simulink model "Sim_PA_DDPG_4drone"  (R2025a)
settings: Solver=ode1  StartTime=0.0  StopTime=Tf  FixedStep=Ts_Sim  RelTol=1e-3
undefined symbols (not defined in the file): control_noise, p_IC, phi_IC, phi_limit, pqr_Limit, psi_dsr, psi_IC, psi_limit, q_IC, r_IC, saturation_logic, state_noise, theta_IC, theta_limit, Ts_Sim, u_IC, uvw_Limit, v_IC, w_IC, wind_logic, x_IC, xy_Limit, y_IC, z_IC, z_Limit
libraries: rllib x8
(part 1 of 2)
settings Model: Creator=nt488543  LastModifiedBy=re606359

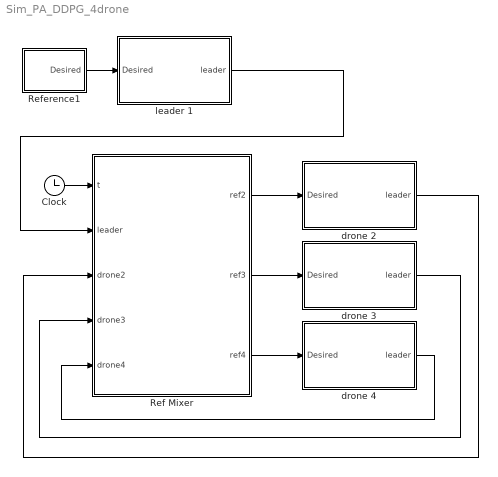
== system Sim_PA_DDPG_4drone ==
  Clock : Clock
  Ref Mixer : MATLAB Function  TreatAsAtomicUnit=on
  Reference1 : Subsystem
  drone 2 : Subsystem
  drone 3 : Subsystem
  drone 4 : Subsystem
  leader 1 : Subsystem
  wires:
  Reference1/1(Desired) -> leader 1/1(Desired)
  Clock/1 -> Ref Mixer/1(t)
  leader 1/1(leader) -> Ref Mixer/2(leader)
  Ref Mixer/1(ref2) -> drone 2/1(Desired)
  Ref Mixer/2(ref3) -> drone 3/1(Desired)
  Ref Mixer/3(ref4) -> drone 4/1(Desired)
  drone 2/1(leader) -> Ref Mixer/3(drone2)
  drone 3/1(leader) -> Ref Mixer/4(drone3)
  drone 4/1(leader) -> Ref Mixer/5(drone4)

== system Sim_PA_DDPG_4drone/Reference1 ==
  Clock1 : Clock
  Mux : Mux  Inputs=6
  Position Reference Signal : MATLAB Function  TreatAsAtomicUnit=on
  To Workspace : ToWorkspace  VariableName=X_ref  SampleTime=Ts_Sim
  Desired : Outport
  wires:
  Position Reference Signal/2(y_desired) -> Mux/2  "y_desired"
  Position Reference Signal/4(xdot_desired) -> Mux/4  "u_desired"
  Position Reference Signal/6(zdot_desired) -> Mux/6  "w_desired"
  Clock1/1 -> Position Reference Signal/1(t)
  Position Reference Signal/3(z_desired) -> Mux/3  "z_desired"
  Position Reference Signal/1(x_desired) -> Mux/1  "x_desired"
  Position Reference Signal/5(ydot_desired) -> Mux/5  "v_desired"
  Mux/1 -> To Workspace/1, Desired/1  "Desired"

== system Sim_PA_DDPG_4drone/drone 2 ==
  note: Inner Loop
  Desired : Inport
  Attitude DDPG : Subsystem
  Drone Dynamics : Subsystem
  Position DDPG : Subsystem
  System Solver : Subsystem
  leader : Outport
  wires:
  Drone Dynamics/2(Actual Angle & its Rate) -> Attitude DDPG/2(Actual Angle)
  System Solver/1(Ang Ref) -> Attitude DDPG/1(Angle Reference)
  Attitude DDPG/1(Tau) -> Drone Dynamics/1(Tau)  "Tau"
  System Solver/2(ft) -> Drone Dynamics/2(ft)
  Desired/1 -> Position DDPG/1(Desired)
  Position DDPG/1(uvw Dot) -> System Solver/1(uvw Dot)
  Drone Dynamics/1(Actual Position & Velocity) -> Position DDPG/2(Actual Position & Velocity), leader/1  "Outer Loop"

== system Sim_PA_DDPG_4drone/drone 3 ==
  note: Inner Loop
  Desired : Inport
  Attitude DDPG : Subsystem
  Drone Dynamics : Subsystem
  Position DDPG : Subsystem
  System Solver : Subsystem
  leader : Outport
  wires:
  Drone Dynamics/1(Actual Position & Velocity) -> leader/1, Position DDPG/2(Actual Position & Velocity)  "Outer Loop"
  Position DDPG/1(uvw Dot) -> System Solver/1(uvw Dot)
  Desired/1 -> Position DDPG/1(Desired)
  System Solver/2(ft) -> Drone Dynamics/2(ft)
  Attitude DDPG/1(Tau) -> Drone Dynamics/1(Tau)  "Tau"
  System Solver/1(Ang Ref) -> Attitude DDPG/1(Angle Reference)
  Drone Dynamics/2(Actual Angle & its Rate) -> Attitude DDPG/2(Actual Angle)

== system Sim_PA_DDPG_4drone/drone 4 ==
  note: Inner Loop
  Desired : Inport
  Attitude DDPG : Subsystem
  Drone Dynamics : Subsystem
  Position DDPG : Subsystem
  System Solver : Subsystem
  leader : Outport
  wires:
  Drone Dynamics/2(Actual Angle & its Rate) -> Attitude DDPG/2(Actual Angle)
  System Solver/1(Ang Ref) -> Attitude DDPG/1(Angle Reference)
  Attitude DDPG/1(Tau) -> Drone Dynamics/1(Tau)  "Tau"
  System Solver/2(ft) -> Drone Dynamics/2(ft)
  Desired/1 -> Position DDPG/1(Desired)
  Position DDPG/1(uvw Dot) -> System Solver/1(uvw Dot)
  Drone Dynamics/1(Actual Position & Velocity) -> Position DDPG/2(Actual Position & Velocity), leader/1  "Outer Loop"

== system Sim_PA_DDPG_4drone/leader 1 ==
  note: Inner Loop
  Desired : Inport
  Attitude DDPG : Subsystem
  Drone Dynamics : Subsystem
  Position DDPG : Subsystem
  System Solver : Subsystem
  leader : Outport
  wires:
  Drone Dynamics/1(Actual Position & Velocity) -> leader/1, Position DDPG/2(Actual Position & Velocity)  "Outer Loop"
  Position DDPG/1(uvw Dot) -> System Solver/1(uvw Dot)
  Desired/1 -> Position DDPG/1(Desired)
  System Solver/2(ft) -> Drone Dynamics/2(ft)
  Attitude DDPG/1(Tau) -> Drone Dynamics/1(Tau)  "Tau"
  System Solver/1(Ang Ref) -> Attitude DDPG/1(Angle Reference)
  Drone Dynamics/2(Actual Angle & its Rate) -> Attitude DDPG/2(Actual Angle)

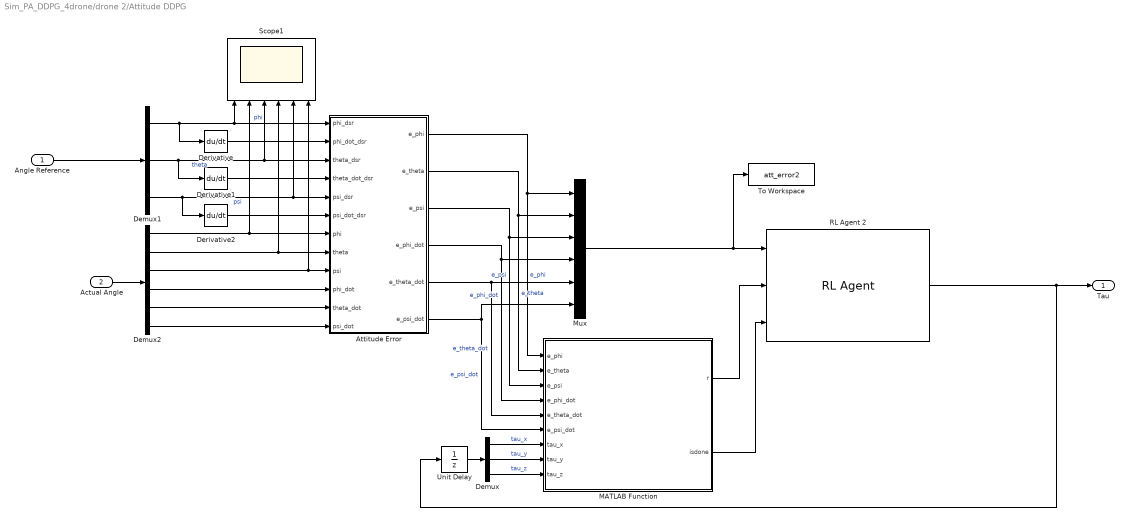
== system Sim_PA_DDPG_4drone/drone 2/Attitude DDPG ==
  Angle Reference : Inport
  Actual Angle : Inport  Port=2
  Attitude Error : MATLAB Function  TreatAsAtomicUnit=on
  Demux : Demux  Outputs=3
  Demux1 : Demux  Outputs=3
  Demux2 : Demux  Outputs=6
  Derivative : Derivative
  Derivative1 : Derivative
  Derivative2 : Derivative
  MATLAB Function : MATLAB Function  TreatAsAtomicUnit=on
  Mux : Mux  Inputs=6
  RL Agent 2 : rllib/RL Agent  Agent=agent2  ExternalActionAsInput=off  ProvideLastAction=off  ProvideCumRwd=off  TreatAsDirectFeedthrough=on  UseStrictObservationDataTypes=off
  Scope1 : Scope  NumInputPorts=6
      settings: ActiveDisplayYMinimum=-0.08548920227975057  ActiveDisplayYMaximum=0.079586119310867051  DataLoggingVariableName=ScopeData6
  To Workspace : ToWorkspace  VariableName=att_error2  SampleTime=Ts_Sim
  Unit Delay : UnitDelay  SampleTime=Ts_Sim  HasFrameUpgradeWarning=on
  Tau : Outport
  wires:
  Derivative2/1 -> Attitude Error/6(psi_dot_dsr)
  Derivative1/1 -> Attitude Error/4(theta_dot_dsr)
  Derivative/1 -> Attitude Error/2(phi_dot_dsr)
  Angle Reference/1 -> Demux1/1
  Demux1/2 -> Scope1/3, Attitude Error/3(theta_dsr), Derivative1/1  "theta"
  Demux1/3 -> Scope1/5, Attitude Error/5(psi_dsr), Derivative2/1  "psi"
  Demux1/1 -> Scope1/1, Attitude Error/1(phi_dsr), Derivative/1  "phi"
  Unit Delay/1 -> Demux/1
  Actual Angle/1 -> Demux2/1
  Demux2/6 -> Attitude Error/12(psi_dot)
  Demux2/5 -> Attitude Error/11(theta_dot)
  Demux2/4 -> Attitude Error/10(phi_dot)
  Demux2/3 -> Scope1/6, Attitude Error/9(psi)
  Demux2/2 -> Attitude Error/8(theta), Scope1/4
  Demux2/1 -> Attitude Error/7(phi), Scope1/2
  RL Agent 2/1 -> Tau/1, Unit Delay/1
  Demux/3 -> MATLAB Function/9(tau_z)  "tau_z"
  Demux/2 -> MATLAB Function/8(tau_y)  "tau_y"
  Demux/1 -> MATLAB Function/7(tau_x)  "tau_x"
  MATLAB Function/2(isdone) -> RL Agent 2/3
  Attitude Error/6(e_psi_dot) -> Mux/6, MATLAB Function/6(e_psi_dot)  "e_psi_dot"
  Attitude Error/5(e_theta_dot) -> Mux/5, MATLAB Function/5(e_theta_dot)  "e_theta_dot"
  Attitude Error/4(e_phi_dot) -> MATLAB Function/4(e_phi_dot), Mux/4  "e_phi_dot"
  Attitude Error/3(e_psi) -> MATLAB Function/3(e_psi), Mux/3  "e_psi"
  Attitude Error/2(e_theta) -> MATLAB Function/2(e_theta), Mux/2  "e_theta"
  Attitude Error/1(e_phi) -> MATLAB Function/1(e_phi), Mux/1  "e_phi"
  Mux/1 -> RL Agent 2/1, To Workspace/1
  MATLAB Function/1(r) -> RL Agent 2/2

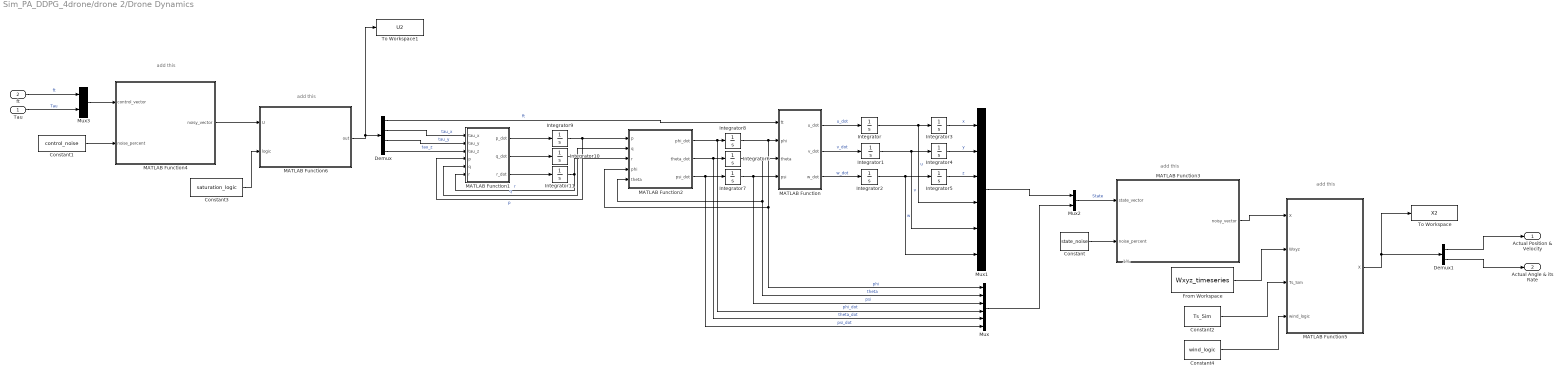
== system Sim_PA_DDPG_4drone/drone 2/Drone Dynamics ==
  note: add this
  note: add this
  note: add this
  note: 1%
  note: add this
  Tau : Inport
  ft : Inport  Port=2
  Constant : Constant  Value=state_noise  SampleTime=Ts_Sim
  Constant1 : Constant  Value=control_noise
  Constant2 : Constant  Value=Ts_Sim
  Constant3 : Constant  Value=saturation_logic  SampleTime=Ts_Sim
  Constant4 : Constant  Value=wind_logic
  Demux : Demux
  Demux1 : Demux  Outputs=2
  From Workspace : FromWorkspace  VariableName=Wxyz_timeseries  SampleTime=Ts_Sim
  Integrator : Integrator  InitialCondition=u_IC  UpperSaturationLimit=uvw_Limit  LowerSaturationLimit=-uvw_Limit
  Integrator1 : Integrator  InitialCondition=v_IC  UpperSaturationLimit=uvw_Limit  LowerSaturationLimit=-uvw_Limit
  Integrator10 : Integrator  InitialCondition=q_IC  UpperSaturationLimit=pqr_Limit  LowerSaturationLimit=-pqr_Limit
  Integrator11 : Integrator  InitialCondition=r_IC  UpperSaturationLimit=pqr_Limit  LowerSaturationLimit=-pqr_Limit
  Integrator2 : Integrator  InitialCondition=w_IC  UpperSaturationLimit=uvw_Limit  LowerSaturationLimit=-uvw_Limit
  Integrator3 : Integrator  InitialCondition=x_IC  UpperSaturationLimit=xy_Limit  LowerSaturationLimit=-xy_Limit
  Integrator4 : Integrator  InitialCondition=y_IC  UpperSaturationLimit=xy_Limit  LowerSaturationLimit=-xy_Limit
  Integrator5 : Integrator  InitialCondition=z_IC  UpperSaturationLimit=z_Limit  LowerSaturationLimit=-z_Limit
  Integrator6 : Integrator  InitialCondition=theta_IC  UpperSaturationLimit=theta_limit  LowerSaturationLimit=-theta_limit  WrappedStateUpperValue=pi/2  WrappedStateLowerValue=-pi/2
  Integrator7 : Integrator  InitialCondition=psi_IC  UpperSaturationLimit=psi_limit  LowerSaturationLimit=-psi_limit
  Integrator8 : Integrator  InitialCondition=phi_IC  UpperSaturationLimit=phi_limit  LowerSaturationLimit=-phi_limit
  Integrator9 : Integrator  InitialCondition=p_IC  UpperSaturationLimit=pqr_Limit  LowerSaturationLimit=-pqr_Limit
  MATLAB Function : MATLAB Function  TreatAsAtomicUnit=on
  MATLAB Function1 : MATLAB Function  TreatAsAtomicUnit=on
  MATLAB Function2 : MATLAB Function  TreatAsAtomicUnit=on
  MATLAB Function3 : MATLAB Function  TreatAsAtomicUnit=on
  MATLAB Function4 : MATLAB Function  TreatAsAtomicUnit=on
  MATLAB Function5 : MATLAB Function  TreatAsAtomicUnit=on
  MATLAB Function6 : MATLAB Function  TreatAsAtomicUnit=on
  Mux : Mux  Inputs=6
  Mux1 : Mux  Inputs=6
  Mux2 : Mux  Inputs=2
  Mux3 : Mux  Inputs=2
  To Workspace : ToWorkspace  VariableName=X2  SampleTime=Ts_Sim
  To Workspace1 : ToWorkspace  VariableName=U2  SampleTime=Ts_Sim
  Actual Position & Velocity : Outport
  Actual Angle & its Rate : Outport  Port=2
  wires:
  Constant4/1 -> MATLAB Function5/4(wind_logic)
  Constant3/1 -> MATLAB Function6/2(logic)
  MATLAB Function6/1(out) -> Demux/1, To Workspace1/1
  MATLAB Function5/1(X) -> Demux1/1, To Workspace/1
  Constant2/1 -> MATLAB Function5/3(Ts_Sim)
  Demux1/1 -> Actual Position & Velocity/1
  Demux1/2 -> Actual Angle & its Rate/1
  From Workspace/1 -> MATLAB Function5/2(Wxyz)
  Demux/1 -> MATLAB Function/1(ft)  "ft"
  MATLAB Function4/1(noisy_vector) -> MATLAB Function6/1(U)
  Constant1/1 -> MATLAB Function4/2(noise_percent)
  Mux3/1 -> MATLAB Function4/1(control_vector)
  Constant/1 -> MATLAB Function3/2(noise_percent)
  Mux1/1 -> Mux2/1
  MATLAB Function3/1(noisy_vector) -> MATLAB Function5/1("X ")
  Mux2/1 -> MATLAB Function3/1(state_vector)  "State"
  MATLAB Function2/3(psi_dot) -> Integrator7/1, Mux/6  "psi_dot"
  MATLAB Function2/2(theta_dot) -> Integrator6/1, Mux/5  "theta_dot"
  MATLAB Function2/1(phi_dot) -> Integrator8/1, Mux/4  "phi_dot"
  Demux/2 -> MATLAB Function1/1(tau_x)  "tau_x"
  MATLAB Function1/2(q_dot) -> Integrator10/1
  MATLAB Function/2(v_dot) -> Integrator1/1  "v_dot"
  MATLAB Function/1(u_dot) -> Integrator/1  "u_dot"
  MATLAB Function/3(w_dot) -> Integrator2/1  "w_dot"
  Mux/1 -> Mux2/2
  Demux/4 -> MATLAB Function1/3(tau_z)  "tau_z"
  Integrator10/1 -> MATLAB Function1/5(q), MATLAB Function2/2(q)  "q"
  Integrator6/1 -> MATLAB Function2/5(theta), Mux/2, MATLAB Function/3(theta)  "theta"
  Integrator8/1 -> MATLAB Function/2(phi), MATLAB Function2/4(phi), Mux/1  "phi"
  Integrator7/1 -> MATLAB Function/4(psi), Mux/3  "psi"
  Tau/1 -> Mux3/2  "Tau"
  Integrator/1 -> Integrator3/1, Mux1/4  "u"
  Integrator2/1 -> Integrator5/1, Mux1/6  "w"
  Integrator11/1 -> MATLAB Function2/3(r), MATLAB Function1/6(r)  "r"
  Integrator9/1 -> MATLAB Function2/1(p), MATLAB Function1/4(p)  "p"
  Demux/3 -> MATLAB Function1/2(tau_y)  "tau_y"
  ft/1 -> Mux3/1  "ft"
  Integrator1/1 -> Integrator4/1, Mux1/5  "v"
  Integrator5/1 -> Mux1/3  "z"
  Integrator3/1 -> Mux1/1  "x"
  MATLAB Function1/1(p_dot) -> Integrator9/1
  MATLAB Function1/3(r_dot) -> Integrator11/1
  Integrator4/1 -> Mux1/2  "y"

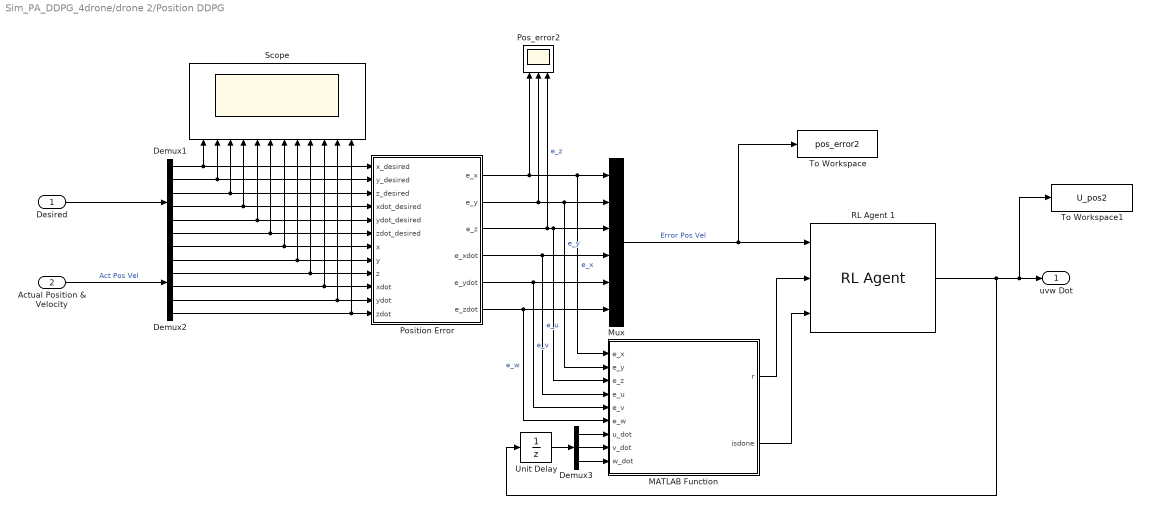
== system Sim_PA_DDPG_4drone/drone 2/Position DDPG ==
  Desired : Inport
  Actual Position & Velocity : Inport  Port=2
  Demux1 : Demux  Outputs=6
  Demux2 : Demux  Outputs=6
  Demux3 : Demux  Outputs=3
  MATLAB Function : MATLAB Function  TreatAsAtomicUnit=on
  Mux : Mux  Inputs=6
  Pos_error2 : Scope  NumInputPorts=3
      settings: ActiveDisplayYMinimum=-19.835443512065805  ActiveDisplayYMaximum=10.081140709923583  DataLoggingVariableName=Error2
  Position Error : MATLAB Function  TreatAsAtomicUnit=on
  RL Agent 1 : rllib/RL Agent  Agent=agent  ExternalActionAsInput=off  ProvideLastAction=off  ProvideCumRwd=off  TreatAsDirectFeedthrough=on  UseStrictObservationDataTypes=off
  Scope : Scope  NumInputPorts=12
      settings: ActiveDisplayYMinimum=-58.33042936718266  ActiveDisplayYMaximum=11.607599309056914  DataLoggingVariableName=Difference
  To Workspace : ToWorkspace  VariableName=pos_error2  SampleTime=Ts_Sim
  To Workspace1 : ToWorkspace  VariableName=U_pos2  SampleTime=Ts_Sim
  Unit Delay : UnitDelay  SampleTime=Ts_Sim  HasFrameUpgradeWarning=on
  uvw Dot : Outport
  wires:
  Unit Delay/1 -> Demux3/1
  Demux3/3 -> MATLAB Function/9(w_dot)
  Demux3/2 -> MATLAB Function/8(v_dot)
  Demux3/1 -> MATLAB Function/7(u_dot)
  Actual Position & Velocity/1 -> Demux2/1  "Act Pos Vel"
  Demux2/6 -> Position Error/12(zdot), Scope/12
  Demux2/5 -> Scope/11, Position Error/11(ydot)
  Demux2/4 -> Scope/10, Position Error/10(xdot)
  Demux2/3 -> Scope/9, Position Error/9(z)
  Demux2/2 -> Scope/8, Position Error/8(y)
  Demux2/1 -> Scope/7, Position Error/7(x)
  Desired/1 -> Demux1/1
  Demux1/6 -> Scope/6, Position Error/6(zdot_desired)
  Demux1/5 -> Scope/5, Position Error/5(ydot_desired)
  Demux1/4 -> Scope/4, Position Error/4(xdot_desired)
  Demux1/3 -> Scope/3, Position Error/3(z_desired)
  Demux1/2 -> Scope/2, Position Error/2(y_desired)
  Demux1/1 -> Scope/1, Position Error/1(x_desired)
  MATLAB Function/2(isdone) -> RL Agent 1/3
  Position Error/6(e_zdot) -> Mux/6, MATLAB Function/6(e_w)  "e_w"
  Position Error/5(e_ydot) -> Mux/5, MATLAB Function/5(e_v)  "e_v"
  Position Error/4(e_xdot) -> Mux/4, MATLAB Function/4(e_u)  "e_u"
  RL Agent 1/1 -> Unit Delay/1, uvw Dot/1, To Workspace1/1
  Mux/1 -> RL Agent 1/1, To Workspace/1  "Error Pos Vel"
  MATLAB Function/1(r) -> RL Agent 1/2
  Position Error/3(e_z) -> Pos_error2/3, MATLAB Function/3(e_z), Mux/3  "e_z"
  Position Error/1(e_x) -> Pos_error2/1, Mux/1, MATLAB Function/1(e_x)  "e_x"
  Position Error/2(e_y) -> Pos_error2/2, Mux/2, MATLAB Function/2(e_y)  "e_y"

== system Sim_PA_DDPG_4drone/drone 2/System Solver ==
  uvw Dot : Inport
  Clock : Clock
  Constant : Constant  Value=psi_dsr
  Demux : Demux  Outputs=3
  Mux : Mux  Inputs=3
  Scope : Scope
      settings: ActiveDisplayYMinimum=5.5477079741609581  ActiveDisplayYMaximum=13.965080226414941
  System Solver : MATLAB Function  TreatAsAtomicUnit=on
  Ang Ref : Outport
  ft : Outport  Port=2
  wires:
  Constant/1 -> System Solver/5("r_yaw ")
  uvw Dot/1 -> Demux/1
  Mux/1 -> Ang Ref/1  "Ang Ref"
  Clock/1 -> System Solver/4(Ts)
  System Solver/4(ft) -> Scope/1, ft/1  "ft"
  Demux/3 -> System Solver/3(u3)
  System Solver/1(roll) -> Mux/1
  Demux/2 -> System Solver/2(u2)
  System Solver/3(r_yaw) -> Mux/3
  Demux/1 -> System Solver/1(u1)
  System Solver/2(pitch) -> Mux/2

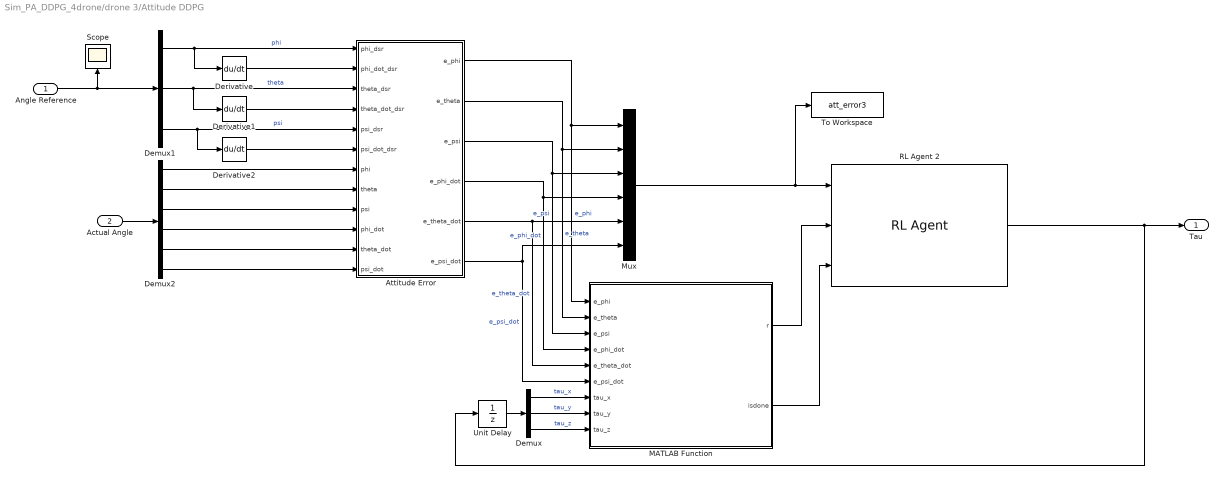
== system Sim_PA_DDPG_4drone/drone 3/Attitude DDPG ==
  Angle Reference : Inport
  Actual Angle : Inport  Port=2
  Attitude Error : MATLAB Function  TreatAsAtomicUnit=on
  Demux : Demux  Outputs=3
  Demux1 : Demux  Outputs=3
  Demux2 : Demux  Outputs=6
  Derivative : Derivative
  Derivative1 : Derivative
  Derivative2 : Derivative
  MATLAB Function : MATLAB Function  TreatAsAtomicUnit=on
  Mux : Mux  Inputs=6
  RL Agent 2 : rllib/RL Agent  Agent=agent2  ExternalActionAsInput=off  ProvideLastAction=off  ProvideCumRwd=off  TreatAsDirectFeedthrough=on  UseStrictObservationDataTypes=off
  Scope : Scope
      settings: ActiveDisplayYMinimum=-0.07573  ActiveDisplayYMaximum=0.06612  DataLoggingVariableName=ScopeData5
  To Workspace : ToWorkspace  VariableName=att_error3  SampleTime=Ts_Sim
  Unit Delay : UnitDelay  SampleTime=Ts_Sim  HasFrameUpgradeWarning=on
  Tau : Outport
  wires:
  MATLAB Function/1(r) -> RL Agent 2/2
  Mux/1 -> To Workspace/1, RL Agent 2/1
  Attitude Error/1(e_phi) -> Mux/1, MATLAB Function/1(e_phi)  "e_phi"
  Attitude Error/2(e_theta) -> Mux/2, MATLAB Function/2(e_theta)  "e_theta"
  Attitude Error/3(e_psi) -> Mux/3, MATLAB Function/3(e_psi)  "e_psi"
  Attitude Error/4(e_phi_dot) -> Mux/4, MATLAB Function/4(e_phi_dot)  "e_phi_dot"
  Attitude Error/5(e_theta_dot) -> MATLAB Function/5(e_theta_dot), Mux/5  "e_theta_dot"
  Attitude Error/6(e_psi_dot) -> MATLAB Function/6(e_psi_dot), Mux/6  "e_psi_dot"
  MATLAB Function/2(isdone) -> RL Agent 2/3
  Demux/1 -> MATLAB Function/7(tau_x)  "tau_x"
  Demux/2 -> MATLAB Function/8(tau_y)  "tau_y"
  Demux/3 -> MATLAB Function/9(tau_z)  "tau_z"
  RL Agent 2/1 -> Unit Delay/1, Tau/1
  Demux2/1 -> Attitude Error/7(phi)
  Demux2/2 -> Attitude Error/8(theta)
  Demux2/3 -> Attitude Error/9(psi)
  Demux2/4 -> Attitude Error/10(phi_dot)
  Demux2/5 -> Attitude Error/11(theta_dot)
  Demux2/6 -> Attitude Error/12(psi_dot)
  Actual Angle/1 -> Demux2/1
  Unit Delay/1 -> Demux/1
  Demux1/1 -> Derivative/1, Attitude Error/1(phi_dsr)  "phi"
  Demux1/3 -> Derivative2/1, Attitude Error/5(psi_dsr)  "psi"
  Demux1/2 -> Derivative1/1, Attitude Error/3(theta_dsr)  "theta"
  Angle Reference/1 -> Demux1/1, Scope/1
  Derivative/1 -> Attitude Error/2(phi_dot_dsr)
  Derivative1/1 -> Attitude Error/4(theta_dot_dsr)
  Derivative2/1 -> Attitude Error/6(psi_dot_dsr)

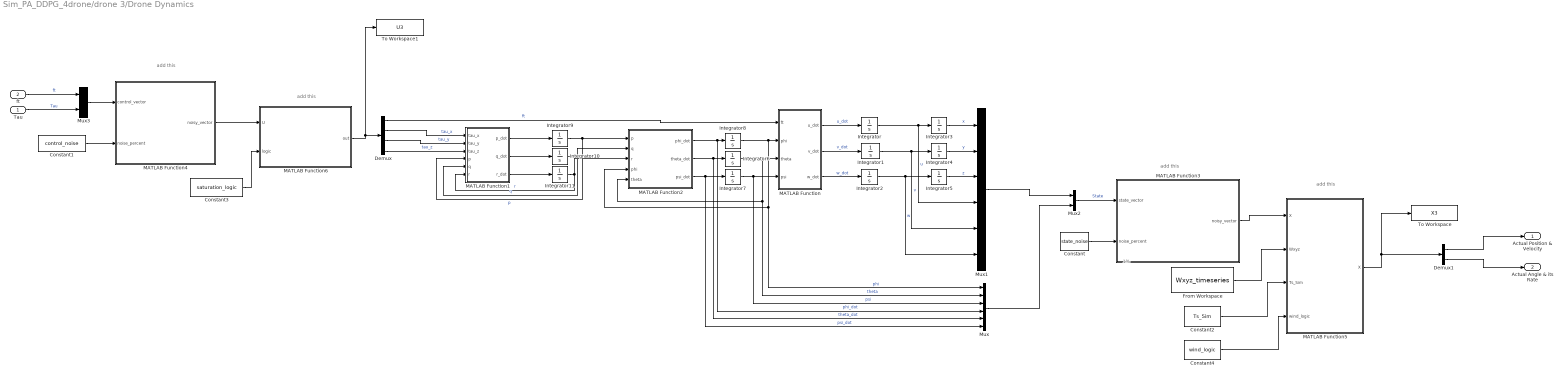
== system Sim_PA_DDPG_4drone/drone 3/Drone Dynamics ==
  note: add this
  note: 1%
  note: add this
  note: add this
  note: add this
  Tau : Inport
  ft : Inport  Port=2
  Constant : Constant  Value=state_noise  SampleTime=Ts_Sim
  Constant1 : Constant  Value=control_noise
  Constant2 : Constant  Value=Ts_Sim
  Constant3 : Constant  Value=saturation_logic  SampleTime=Ts_Sim
  Constant4 : Constant  Value=wind_logic
  Demux : Demux
  Demux1 : Demux  Outputs=2
  From Workspace : FromWorkspace  VariableName=Wxyz_timeseries  SampleTime=Ts_Sim
  Integrator : Integrator  InitialCondition=u_IC  UpperSaturationLimit=uvw_Limit  LowerSaturationLimit=-uvw_Limit
  Integrator1 : Integrator  InitialCondition=v_IC  UpperSaturationLimit=uvw_Limit  LowerSaturationLimit=-uvw_Limit
  Integrator10 : Integrator  InitialCondition=q_IC  UpperSaturationLimit=pqr_Limit  LowerSaturationLimit=-pqr_Limit
  Integrator11 : Integrator  InitialCondition=r_IC  UpperSaturationLimit=pqr_Limit  LowerSaturationLimit=-pqr_Limit
  Integrator2 : Integrator  InitialCondition=w_IC  UpperSaturationLimit=uvw_Limit  LowerSaturationLimit=-uvw_Limit
  Integrator3 : Integrator  InitialCondition=x_IC  UpperSaturationLimit=xy_Limit  LowerSaturationLimit=-xy_Limit
  Integrator4 : Integrator  InitialCondition=y_IC  UpperSaturationLimit=xy_Limit  LowerSaturationLimit=-xy_Limit
  Integrator5 : Integrator  InitialCondition=z_IC  UpperSaturationLimit=z_Limit  LowerSaturationLimit=-z_Limit
  Integrator6 : Integrator  InitialCondition=theta_IC  UpperSaturationLimit=theta_limit  LowerSaturationLimit=-theta_limit  WrappedStateUpperValue=pi/2  WrappedStateLowerValue=-pi/2
  Integrator7 : Integrator  InitialCondition=psi_IC  UpperSaturationLimit=psi_limit  LowerSaturationLimit=-psi_limit
  Integrator8 : Integrator  InitialCondition=phi_IC  UpperSaturationLimit=phi_limit  LowerSaturationLimit=-phi_limit
  Integrator9 : Integrator  InitialCondition=p_IC  UpperSaturationLimit=pqr_Limit  LowerSaturationLimit=-pqr_Limit
  MATLAB Function : MATLAB Function  TreatAsAtomicUnit=on
  MATLAB Function1 : MATLAB Function  TreatAsAtomicUnit=on
  MATLAB Function2 : MATLAB Function  TreatAsAtomicUnit=on
  MATLAB Function3 : MATLAB Function  TreatAsAtomicUnit=on
  MATLAB Function4 : MATLAB Function  TreatAsAtomicUnit=on
  MATLAB Function5 : MATLAB Function  TreatAsAtomicUnit=on
  MATLAB Function6 : MATLAB Function  TreatAsAtomicUnit=on
  Mux : Mux  Inputs=6
  Mux1 : Mux  Inputs=6
  Mux2 : Mux  Inputs=2
  Mux3 : Mux  Inputs=2
  To Workspace : ToWorkspace  VariableName=X3  SampleTime=Ts_Sim
  To Workspace1 : ToWorkspace  VariableName=U3  SampleTime=Ts_Sim
  Actual Position & Velocity : Outport
  Actual Angle & its Rate : Outport  Port=2
  wires:
  Integrator4/1 -> Mux1/2  "y"
  MATLAB Function1/3(r_dot) -> Integrator11/1
  MATLAB Function1/1(p_dot) -> Integrator9/1
  Integrator3/1 -> Mux1/1  "x"
  Integrator5/1 -> Mux1/3  "z"
  Integrator1/1 -> Mux1/5, Integrator4/1  "v"
  ft/1 -> Mux3/1  "ft"
  Demux/3 -> MATLAB Function1/2(tau_y)  "tau_y"
  Integrator9/1 -> MATLAB Function1/4(p), MATLAB Function2/1(p)  "p"
  Integrator11/1 -> MATLAB Function1/6(r), MATLAB Function2/3(r)  "r"
  Integrator2/1 -> Mux1/6, Integrator5/1  "w"
  Integrator/1 -> Mux1/4, Integrator3/1  "u"
  Tau/1 -> Mux3/2  "Tau"
  Integrator7/1 -> Mux/3, MATLAB Function/4(psi)  "psi"
  Integrator8/1 -> Mux/1, MATLAB Function2/4(phi), MATLAB Function/2(phi)  "phi"
  Integrator6/1 -> MATLAB Function/3(theta), Mux/2, MATLAB Function2/5(theta)  "theta"
  Integrator10/1 -> MATLAB Function2/2(q), MATLAB Function1/5(q)  "q"
  Demux/4 -> MATLAB Function1/3(tau_z)  "tau_z"
  Mux/1 -> Mux2/2
  MATLAB Function/3(w_dot) -> Integrator2/1  "w_dot"
  MATLAB Function/1(u_dot) -> Integrator/1  "u_dot"
  MATLAB Function/2(v_dot) -> Integrator1/1  "v_dot"
  MATLAB Function1/2(q_dot) -> Integrator10/1
  Demux/2 -> MATLAB Function1/1(tau_x)  "tau_x"
  MATLAB Function2/1(phi_dot) -> Mux/4, Integrator8/1  "phi_dot"
  MATLAB Function2/2(theta_dot) -> Mux/5, Integrator6/1  "theta_dot"
  MATLAB Function2/3(psi_dot) -> Mux/6, Integrator7/1  "psi_dot"
  Mux2/1 -> MATLAB Function3/1(state_vector)  "State"
  MATLAB Function3/1(noisy_vector) -> MATLAB Function5/1("X ")
  Mux1/1 -> Mux2/1
  Constant/1 -> MATLAB Function3/2(noise_percent)
  Mux3/1 -> MATLAB Function4/1(control_vector)
  Constant1/1 -> MATLAB Function4/2(noise_percent)
  MATLAB Function4/1(noisy_vector) -> MATLAB Function6/1(U)
  Demux/1 -> MATLAB Function/1(ft)  "ft"
  From Workspace/1 -> MATLAB Function5/2(Wxyz)
  Demux1/2 -> Actual Angle & its Rate/1
  Demux1/1 -> Actual Position & Velocity/1
  Constant2/1 -> MATLAB Function5/3(Ts_Sim)
  MATLAB Function5/1(X) -> To Workspace/1, Demux1/1
  MATLAB Function6/1(out) -> To Workspace1/1, Demux/1
  Constant3/1 -> MATLAB Function6/2(logic)
  Constant4/1 -> MATLAB Function5/4(wind_logic)

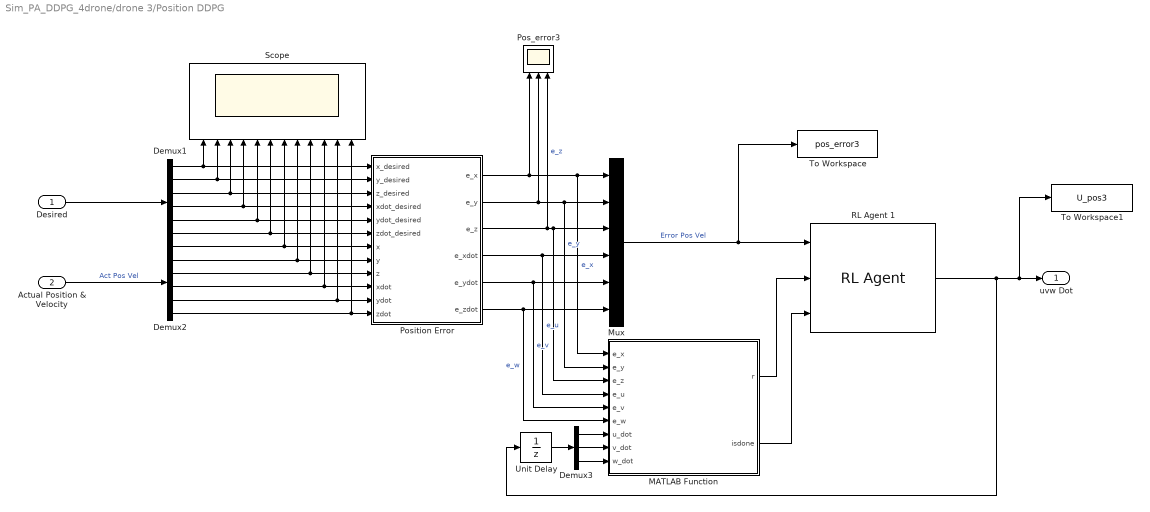
== system Sim_PA_DDPG_4drone/drone 3/Position DDPG ==
  Desired : Inport
  Actual Position & Velocity : Inport  Port=2
  Demux1 : Demux  Outputs=6
  Demux2 : Demux  Outputs=6
  Demux3 : Demux  Outputs=3
  MATLAB Function : MATLAB Function  TreatAsAtomicUnit=on
  Mux : Mux  Inputs=6
  Pos_error3 : Scope  NumInputPorts=3
      settings: ActiveDisplayYMinimum=-26.259185565275498  ActiveDisplayYMaximum=15.642824664105513  DataLoggingVariableName=Error3
  Position Error : MATLAB Function  TreatAsAtomicUnit=on
  RL Agent 1 : rllib/RL Agent  Agent=agent  ExternalActionAsInput=off  ProvideLastAction=off  ProvideCumRwd=off  TreatAsDirectFeedthrough=on  UseStrictObservationDataTypes=off
  Scope : Scope  NumInputPorts=12
      settings: ActiveDisplayYMinimum=-64.8105630976365  ActiveDisplayYMaximum=12.296113517917625  DataLoggingVariableName=Difference
  To Workspace : ToWorkspace  VariableName=pos_error3  SampleTime=Ts_Sim
  To Workspace1 : ToWorkspace  VariableName=U_pos3  SampleTime=Ts_Sim
  Unit Delay : UnitDelay  SampleTime=Ts_Sim  HasFrameUpgradeWarning=on
  uvw Dot : Outport
  wires:
  MATLAB Function/1(r) -> RL Agent 1/2
  Mux/1 -> To Workspace/1, RL Agent 1/1  "Error Pos Vel"
  RL Agent 1/1 -> To Workspace1/1, uvw Dot/1, Unit Delay/1
  Position Error/4(e_xdot) -> MATLAB Function/4(e_u), Mux/4  "e_u"
  Position Error/5(e_ydot) -> MATLAB Function/5(e_v), Mux/5  "e_v"
  Position Error/6(e_zdot) -> MATLAB Function/6(e_w), Mux/6  "e_w"
  MATLAB Function/2(isdone) -> RL Agent 1/3
  Demux1/1 -> Position Error/1(x_desired), Scope/1
  Demux1/2 -> Position Error/2(y_desired), Scope/2
  Demux1/3 -> Position Error/3(z_desired), Scope/3
  Demux1/4 -> Position Error/4(xdot_desired), Scope/4
  Demux1/5 -> Position Error/5(ydot_desired), Scope/5
  Demux1/6 -> Position Error/6(zdot_desired), Scope/6
  Desired/1 -> Demux1/1
  Demux2/1 -> Position Error/7(x), Scope/7
  Demux2/2 -> Position Error/8(y), Scope/8
  Demux2/3 -> Position Error/9(z), Scope/9
  Demux2/4 -> Position Error/10(xdot), Scope/10
  Demux2/5 -> Position Error/11(ydot), Scope/11
  Demux2/6 -> Scope/12, Position Error/12(zdot)
  Actual Position & Velocity/1 -> Demux2/1  "Act Pos Vel"
  Demux3/1 -> MATLAB Function/7(u_dot)
  Demux3/2 -> MATLAB Function/8(v_dot)
  Demux3/3 -> MATLAB Function/9(w_dot)
  Unit Delay/1 -> Demux3/1
  Position Error/3(e_z) -> Pos_error3/3, Mux/3, MATLAB Function/3(e_z)  "e_z"
  Position Error/1(e_x) -> Pos_error3/1, MATLAB Function/1(e_x), Mux/1  "e_x"
  Position Error/2(e_y) -> Pos_error3/2, MATLAB Function/2(e_y), Mux/2  "e_y"

== system Sim_PA_DDPG_4drone/drone 3/System Solver ==
  uvw Dot : Inport
  Clock : Clock
  Constant : Constant  Value=psi_dsr
  Demux : Demux  Outputs=3
  Mux : Mux  Inputs=3
  Scope : Scope
      settings: ActiveDisplayYMinimum=5.5477079741609581  ActiveDisplayYMaximum=13.965080226414941
  System Solver : MATLAB Function  TreatAsAtomicUnit=on
  Ang Ref : Outport
  ft : Outport  Port=2
  wires:
  System Solver/2(pitch) -> Mux/2
  Demux/1 -> System Solver/1(u1)
  System Solver/3(r_yaw) -> Mux/3
  Demux/2 -> System Solver/2(u2)
  System Solver/1(roll) -> Mux/1
  Demux/3 -> System Solver/3(u3)
  System Solver/4(ft) -> ft/1, Scope/1  "ft"
  Clock/1 -> System Solver/4(Ts)
  Mux/1 -> Ang Ref/1  "Ang Ref"
  uvw Dot/1 -> Demux/1
  Constant/1 -> System Solver/5("r_yaw ")

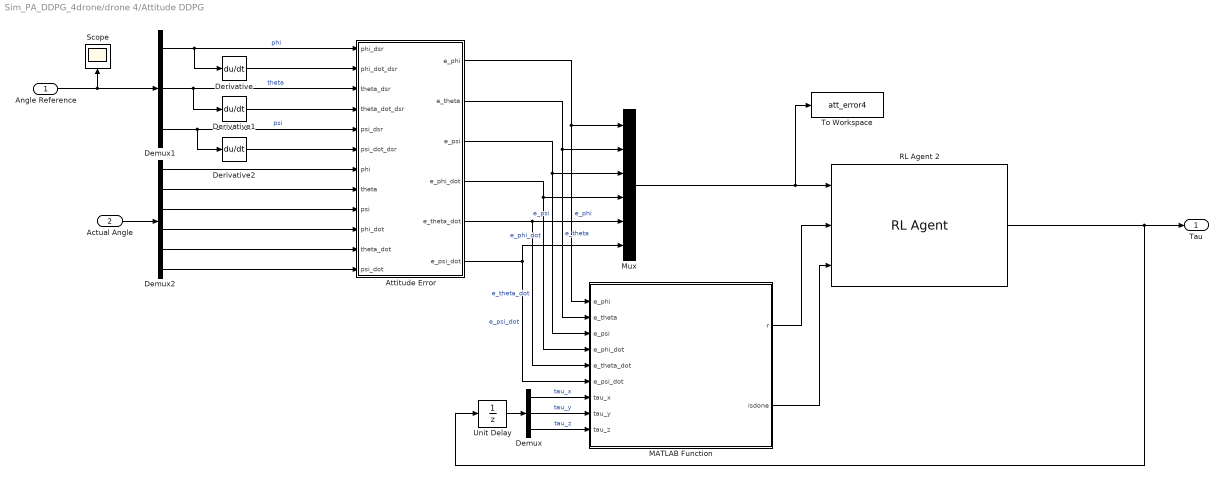
== system Sim_PA_DDPG_4drone/drone 4/Attitude DDPG ==
  Angle Reference : Inport
  Actual Angle : Inport  Port=2
  Attitude Error : MATLAB Function  TreatAsAtomicUnit=on
  Demux : Demux  Outputs=3
  Demux1 : Demux  Outputs=3
  Demux2 : Demux  Outputs=6
  Derivative : Derivative
  Derivative1 : Derivative
  Derivative2 : Derivative
  MATLAB Function : MATLAB Function  TreatAsAtomicUnit=on
  Mux : Mux  Inputs=6
  RL Agent 2 : rllib/RL Agent  Agent=agent2  ExternalActionAsInput=off  ProvideLastAction=off  ProvideCumRwd=off  TreatAsDirectFeedthrough=on  UseStrictObservationDataTypes=off
  Scope : Scope
      settings: ActiveDisplayYMinimum=-0.07573  ActiveDisplayYMaximum=0.06612  DataLoggingVariableName=ScopeData5
  To Workspace : ToWorkspace  VariableName=att_error4  SampleTime=Ts_Sim
  Unit Delay : UnitDelay  SampleTime=Ts_Sim  HasFrameUpgradeWarning=on
  Tau : Outport
  wires:
  Derivative2/1 -> Attitude Error/6(psi_dot_dsr)
  Derivative1/1 -> Attitude Error/4(theta_dot_dsr)
  Derivative/1 -> Attitude Error/2(phi_dot_dsr)
  Angle Reference/1 -> Scope/1, Demux1/1
  Demux1/2 -> Attitude Error/3(theta_dsr), Derivative1/1  "theta"
  Demux1/3 -> Attitude Error/5(psi_dsr), Derivative2/1  "psi"
  Demux1/1 -> Attitude Error/1(phi_dsr), Derivative/1  "phi"
  Unit Delay/1 -> Demux/1
  Actual Angle/1 -> Demux2/1
  Demux2/6 -> Attitude Error/12(psi_dot)
  Demux2/5 -> Attitude Error/11(theta_dot)
  Demux2/4 -> Attitude Error/10(phi_dot)
  Demux2/3 -> Attitude Error/9(psi)
  Demux2/2 -> Attitude Error/8(theta)
  Demux2/1 -> Attitude Error/7(phi)
  RL Agent 2/1 -> Tau/1, Unit Delay/1
  Demux/3 -> MATLAB Function/9(tau_z)  "tau_z"
  Demux/2 -> MATLAB Function/8(tau_y)  "tau_y"
  Demux/1 -> MATLAB Function/7(tau_x)  "tau_x"
  MATLAB Function/2(isdone) -> RL Agent 2/3
  Attitude Error/6(e_psi_dot) -> Mux/6, MATLAB Function/6(e_psi_dot)  "e_psi_dot"
  Attitude Error/5(e_theta_dot) -> Mux/5, MATLAB Function/5(e_theta_dot)  "e_theta_dot"
  Attitude Error/4(e_phi_dot) -> MATLAB Function/4(e_phi_dot), Mux/4  "e_phi_dot"
  Attitude Error/3(e_psi) -> MATLAB Function/3(e_psi), Mux/3  "e_psi"
  Attitude Error/2(e_theta) -> MATLAB Function/2(e_theta), Mux/2  "e_theta"
  Attitude Error/1(e_phi) -> MATLAB Function/1(e_phi), Mux/1  "e_phi"
  Mux/1 -> RL Agent 2/1, To Workspace/1
  MATLAB Function/1(r) -> RL Agent 2/2

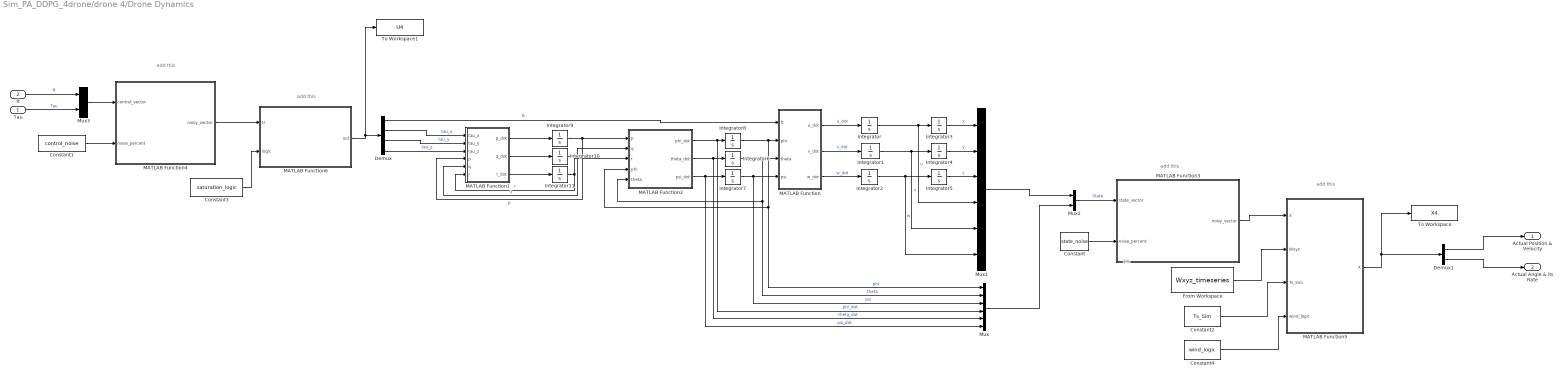
== system Sim_PA_DDPG_4drone/drone 4/Drone Dynamics ==
  note: add this
  note: add this
  note: add this
  note: 1%
  note: add this
  Tau : Inport
  ft : Inport  Port=2
  Constant : Constant  Value=state_noise  SampleTime=Ts_Sim
  Constant1 : Constant  Value=control_noise
  Constant2 : Constant  Value=Ts_Sim
  Constant3 : Constant  Value=saturation_logic  SampleTime=Ts_Sim
  Constant4 : Constant  Value=wind_logic
  Demux : Demux
  Demux1 : Demux  Outputs=2
  From Workspace : FromWorkspace  VariableName=Wxyz_timeseries  SampleTime=Ts_Sim
  Integrator : Integrator  InitialCondition=u_IC  UpperSaturationLimit=uvw_Limit  LowerSaturationLimit=-uvw_Limit
  Integrator1 : Integrator  InitialCondition=v_IC  UpperSaturationLimit=uvw_Limit  LowerSaturationLimit=-uvw_Limit
  Integrator10 : Integrator  InitialCondition=q_IC  UpperSaturationLimit=pqr_Limit  LowerSaturationLimit=-pqr_Limit
  Integrator11 : Integrator  InitialCondition=r_IC  UpperSaturationLimit=pqr_Limit  LowerSaturationLimit=-pqr_Limit
  Integrator2 : Integrator  InitialCondition=w_IC  UpperSaturationLimit=uvw_Limit  LowerSaturationLimit=-uvw_Limit
  Integrator3 : Integrator  InitialCondition=x_IC  UpperSaturationLimit=xy_Limit  LowerSaturationLimit=-xy_Limit
  Integrator4 : Integrator  InitialCondition=y_IC  UpperSaturationLimit=xy_Limit  LowerSaturationLimit=-xy_Limit
  Integrator5 : Integrator  InitialCondition=z_IC  UpperSaturationLimit=z_Limit  LowerSaturationLimit=-z_Limit
  Integrator6 : Integrator  InitialCondition=theta_IC  UpperSaturationLimit=theta_limit  LowerSaturationLimit=-theta_limit  WrappedStateUpperValue=pi/2  WrappedStateLowerValue=-pi/2
  Integrator7 : Integrator  InitialCondition=psi_IC  UpperSaturationLimit=psi_limit  LowerSaturationLimit=-psi_limit
  Integrator8 : Integrator  InitialCondition=phi_IC  UpperSaturationLimit=phi_limit  LowerSaturationLimit=-phi_limit
  Integrator9 : Integrator  InitialCondition=p_IC  UpperSaturationLimit=pqr_Limit  LowerSaturationLimit=-pqr_Limit
  MATLAB Function : MATLAB Function  TreatAsAtomicUnit=on
  MATLAB Function1 : MATLAB Function  TreatAsAtomicUnit=on
  MATLAB Function2 : MATLAB Function  TreatAsAtomicUnit=on
  MATLAB Function3 : MATLAB Function  TreatAsAtomicUnit=on
  MATLAB Function4 : MATLAB Function  TreatAsAtomicUnit=on
  MATLAB Function5 : MATLAB Function  TreatAsAtomicUnit=on
  MATLAB Function6 : MATLAB Function  TreatAsAtomicUnit=on
  Mux : Mux  Inputs=6
  Mux1 : Mux  Inputs=6
  Mux2 : Mux  Inputs=2
  Mux3 : Mux  Inputs=2
  To Workspace : ToWorkspace  VariableName=X4  SampleTime=Ts_Sim
  To Workspace1 : ToWorkspace  VariableName=U4  SampleTime=Ts_Sim
  Actual Position & Velocity : Outport
  Actual Angle & its Rate : Outport  Port=2
  wires:
  Constant4/1 -> MATLAB Function5/4(wind_logic)
  Constant3/1 -> MATLAB Function6/2(logic)
  MATLAB Function6/1(out) -> Demux/1, To Workspace1/1
  MATLAB Function5/1(X) -> Demux1/1, To Workspace/1
  Constant2/1 -> MATLAB Function5/3(Ts_Sim)
  Demux1/1 -> Actual Position & Velocity/1
  Demux1/2 -> Actual Angle & its Rate/1
  From Workspace/1 -> MATLAB Function5/2(Wxyz)
  Demux/1 -> MATLAB Function/1(ft)  "ft"
  MATLAB Function4/1(noisy_vector) -> MATLAB Function6/1(U)
  Constant1/1 -> MATLAB Function4/2(noise_percent)
  Mux3/1 -> MATLAB Function4/1(control_vector)
  Constant/1 -> MATLAB Function3/2(noise_percent)
  Mux1/1 -> Mux2/1
  MATLAB Function3/1(noisy_vector) -> MATLAB Function5/1("X ")
  Mux2/1 -> MATLAB Function3/1(state_vector)  "State"
  MATLAB Function2/3(psi_dot) -> Integrator7/1, Mux/6  "psi_dot"
  MATLAB Function2/2(theta_dot) -> Integrator6/1, Mux/5  "theta_dot"
  MATLAB Function2/1(phi_dot) -> Integrator8/1, Mux/4  "phi_dot"
  Demux/2 -> MATLAB Function1/1(tau_x)  "tau_x"
  MATLAB Function1/2(q_dot) -> Integrator10/1
  MATLAB Function/2(v_dot) -> Integrator1/1  "v_dot"
  MATLAB Function/1(u_dot) -> Integrator/1  "u_dot"
  MATLAB Function/3(w_dot) -> Integrator2/1  "w_dot"
  Mux/1 -> Mux2/2
  Demux/4 -> MATLAB Function1/3(tau_z)  "tau_z"
  Integrator10/1 -> MATLAB Function1/5(q), MATLAB Function2/2(q)  "q"
  Integrator6/1 -> MATLAB Function2/5(theta), Mux/2, MATLAB Function/3(theta)  "theta"
  Integrator8/1 -> MATLAB Function/2(phi), MATLAB Function2/4(phi), Mux/1  "phi"
  Integrator7/1 -> MATLAB Function/4(psi), Mux/3  "psi"
  Tau/1 -> Mux3/2  "Tau"
  Integrator/1 -> Integrator3/1, Mux1/4  "u"
  Integrator2/1 -> Integrator5/1, Mux1/6  "w"
  Integrator11/1 -> MATLAB Function2/3(r), MATLAB Function1/6(r)  "r"
  Integrator9/1 -> MATLAB Function2/1(p), MATLAB Function1/4(p)  "p"
  Demux/3 -> MATLAB Function1/2(tau_y)  "tau_y"
  ft/1 -> Mux3/1  "ft"
  Integrator1/1 -> Integrator4/1, Mux1/5  "v"
  Integrator5/1 -> Mux1/3  "z"
  Integrator3/1 -> Mux1/1  "x"
  MATLAB Function1/1(p_dot) -> Integrator9/1
  MATLAB Function1/3(r_dot) -> Integrator11/1
  Integrator4/1 -> Mux1/2  "y"

== system Sim_PA_DDPG_4drone/drone 4/Position DDPG ==
  Desired : Inport
  Actual Position & Velocity : Inport  Port=2
  Demux1 : Demux  Outputs=6
  Demux2 : Demux  Outputs=6
  Demux3 : Demux  Outputs=3
  MATLAB Function : MATLAB Function  TreatAsAtomicUnit=on
  Mux : Mux  Inputs=6
  Pos_error4 : Scope  NumInputPorts=3
      settings: ActiveDisplayYMinimum=-28.66228143189889  ActiveDisplayYMaximum=12.066117124790058  DataLoggingVariableName=Error4
  Position Error : MATLAB Function  TreatAsAtomicUnit=on
  RL Agent 1 : rllib/RL Agent  Agent=agent  ExternalActionAsInput=off  ProvideLastAction=off  ProvideCumRwd=off  TreatAsDirectFeedthrough=on  UseStrictObservationDataTypes=off
  Scope : Scope  NumInputPorts=12
      settings: ActiveDisplayYMinimum=-64.8105630976365  ActiveDisplayYMaximum=12.296113517917625  DataLoggingVariableName=Difference
  To Workspace : ToWorkspace  VariableName=pos_error4  SampleTime=Ts_Sim
  To Workspace1 : ToWorkspace  VariableName=U_pos4  SampleTime=Ts_Sim
  Unit Delay : UnitDelay  SampleTime=Ts_Sim  HasFrameUpgradeWarning=on
  uvw Dot : Outport
  wires:
  Unit Delay/1 -> Demux3/1
  Demux3/3 -> MATLAB Function/9(w_dot)
  Demux3/2 -> MATLAB Function/8(v_dot)
  Demux3/1 -> MATLAB Function/7(u_dot)
  Actual Position & Velocity/1 -> Demux2/1  "Act Pos Vel"
  Demux2/6 -> Position Error/12(zdot), Scope/12
  Demux2/5 -> Scope/11, Position Error/11(ydot)
  Demux2/4 -> Scope/10, Position Error/10(xdot)
  Demux2/3 -> Scope/9, Position Error/9(z)
  Demux2/2 -> Scope/8, Position Error/8(y)
  Demux2/1 -> Scope/7, Position Error/7(x)
  Desired/1 -> Demux1/1
  Demux1/6 -> Scope/6, Position Error/6(zdot_desired)
  Demux1/5 -> Scope/5, Position Error/5(ydot_desired)
  Demux1/4 -> Scope/4, Position Error/4(xdot_desired)
  Demux1/3 -> Scope/3, Position Error/3(z_desired)
  Demux1/2 -> Scope/2, Position Error/2(y_desired)
  Demux1/1 -> Scope/1, Position Error/1(x_desired)
  MATLAB Function/2(isdone) -> RL Agent 1/3
  Position Error/6(e_zdot) -> Mux/6, MATLAB Function/6(e_w)  "e_w"
  Position Error/5(e_ydot) -> Mux/5, MATLAB Function/5(e_v)  "e_v"
  Position Error/4(e_xdot) -> Mux/4, MATLAB Function/4(e_u)  "e_u"
  RL Agent 1/1 -> Unit Delay/1, uvw Dot/1, To Workspace1/1
  Mux/1 -> RL Agent 1/1, To Workspace/1  "Error Pos Vel"
  MATLAB Function/1(r) -> RL Agent 1/2
  Position Error/3(e_z) -> Pos_error4/3, MATLAB Function/3(e_z), Mux/3  "e_z"
  Position Error/1(e_x) -> Pos_error4/1, Mux/1, MATLAB Function/1(e_x)  "e_x"
  Position Error/2(e_y) -> Pos_error4/2, Mux/2, MATLAB Function/2(e_y)  "e_y"

== system Sim_PA_DDPG_4drone/drone 4/System Solver ==
  uvw Dot : Inport
  Clock : Clock
  Constant : Constant  Value=psi_dsr
  Demux : Demux  Outputs=3
  Mux : Mux  Inputs=3
  Scope : Scope
      settings: ActiveDisplayYMinimum=5.5477079741609581  ActiveDisplayYMaximum=13.965080226414941
  System Solver : MATLAB Function  TreatAsAtomicUnit=on
  Ang Ref : Outport
  ft : Outport  Port=2
  wires:
  Constant/1 -> System Solver/5("r_yaw ")
  uvw Dot/1 -> Demux/1
  Mux/1 -> Ang Ref/1  "Ang Ref"
  Clock/1 -> System Solver/4(Ts)
  System Solver/4(ft) -> Scope/1, ft/1  "ft"
  Demux/3 -> System Solver/3(u3)
  System Solver/1(roll) -> Mux/1
  Demux/2 -> System Solver/2(u2)
  System Solver/3(r_yaw) -> Mux/3
  Demux/1 -> System Solver/1(u1)
  System Solver/2(pitch) -> Mux/2

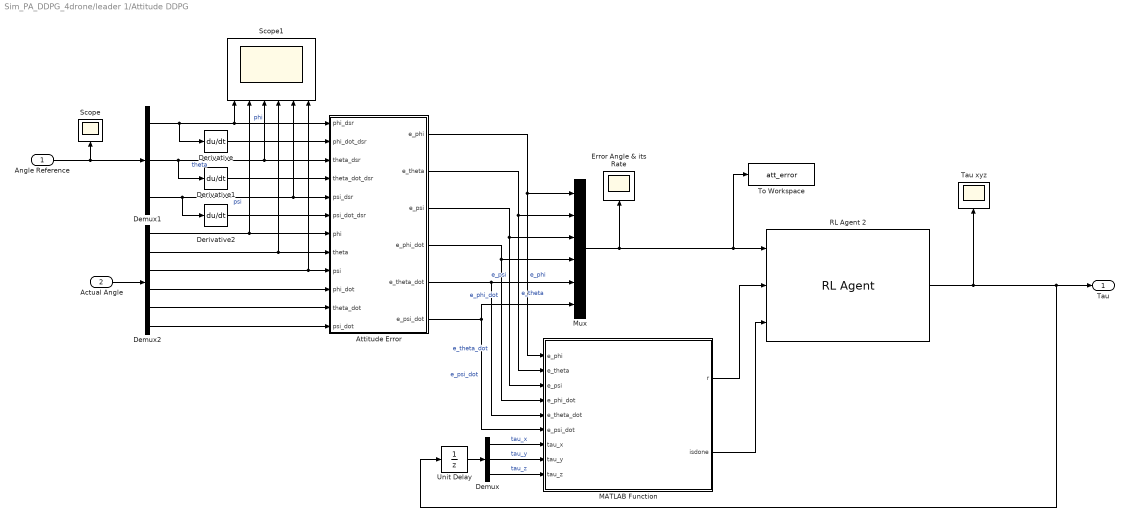
== system Sim_PA_DDPG_4drone/leader 1/Attitude DDPG ==
  Angle Reference : Inport
  Actual Angle : Inport  Port=2
  Attitude Error : MATLAB Function  TreatAsAtomicUnit=on
  Demux : Demux  Outputs=3
  Demux1 : Demux  Outputs=3
  Demux2 : Demux  Outputs=6
  Derivative : Derivative
  Derivative1 : Derivative
  Derivative2 : Derivative
  Error Angle & its Rate : Scope
      settings: ActiveDisplayYMinimum=-3.5181599273654109  ActiveDisplayYMaximum=2.1435969273697308  DataLoggingVariableName=ScopeData12
  MATLAB Function : MATLAB Function  TreatAsAtomicUnit=on
  Mux : Mux  Inputs=6
  RL Agent 2 : rllib/RL Agent  Agent=agent2  ExternalActionAsInput=off  ProvideLastAction=off  ProvideCumRwd=off  TreatAsDirectFeedthrough=on  UseStrictObservationDataTypes=off
  Scope : Scope
      settings: ActiveDisplayYMinimum=-0.07573  ActiveDisplayYMaximum=0.06612  DataLoggingVariableName=ScopeData5
  Scope1 : Scope  NumInputPorts=6
      settings: ActiveDisplayYMinimum=-0.08548920227975057  ActiveDisplayYMaximum=0.079586119310867051  DataLoggingVariableName=ScopeData6
  Tau xyz : Scope
      settings: ActiveDisplayYMinimum=-2.4987406879663467  ActiveDisplayYMaximum=2.4991613775491714  DataLoggingVariableName=ScopeData11
  To Workspace : ToWorkspace  VariableName=att_error  SampleTime=Ts_Sim
  Unit Delay : UnitDelay  SampleTime=Ts_Sim  HasFrameUpgradeWarning=on
  Tau : Outport
  wires:
  MATLAB Function/1(r) -> RL Agent 2/2
  Mux/1 -> To Workspace/1, RL Agent 2/1, Error Angle & its Rate/1
  Attitude Error/1(e_phi) -> Mux/1, MATLAB Function/1(e_phi)  "e_phi"
  Attitude Error/2(e_theta) -> Mux/2, MATLAB Function/2(e_theta)  "e_theta"
  Attitude Error/3(e_psi) -> Mux/3, MATLAB Function/3(e_psi)  "e_psi"
  Attitude Error/4(e_phi_dot) -> Mux/4, MATLAB Function/4(e_phi_dot)  "e_phi_dot"
  Attitude Error/5(e_theta_dot) -> MATLAB Function/5(e_theta_dot), Mux/5  "e_theta_dot"
  Attitude Error/6(e_psi_dot) -> MATLAB Function/6(e_psi_dot), Mux/6  "e_psi_dot"
  MATLAB Function/2(isdone) -> RL Agent 2/3
  Demux/1 -> MATLAB Function/7(tau_x)  "tau_x"
  Demux/2 -> MATLAB Function/8(tau_y)  "tau_y"
  Demux/3 -> MATLAB Function/9(tau_z)  "tau_z"
  RL Agent 2/1 -> Unit Delay/1, Tau/1, Tau xyz/1
  Demux2/1 -> Scope1/2, Attitude Error/7(phi)
  Demux2/2 -> Scope1/4, Attitude Error/8(theta)
  Demux2/3 -> Attitude Error/9(psi), Scope1/6
  Demux2/4 -> Attitude Error/10(phi_dot)
  Demux2/5 -> Attitude Error/11(theta_dot)
  Demux2/6 -> Attitude Error/12(psi_dot)
  Actual Angle/1 -> Demux2/1
  Unit Delay/1 -> Demux/1
  Demux1/1 -> Derivative/1, Attitude Error/1(phi_dsr), Scope1/1  "phi"
  Demux1/3 -> Derivative2/1, Attitude Error/5(psi_dsr), Scope1/5  "psi"
  Demux1/2 -> Derivative1/1, Attitude Error/3(theta_dsr), Scope1/3  "theta"
  Angle Reference/1 -> Demux1/1, Scope/1
  Derivative/1 -> Attitude Error/2(phi_dot_dsr)
  Derivative1/1 -> Attitude Error/4(theta_dot_dsr)
  Derivative2/1 -> Attitude Error/6(psi_dot_dsr)

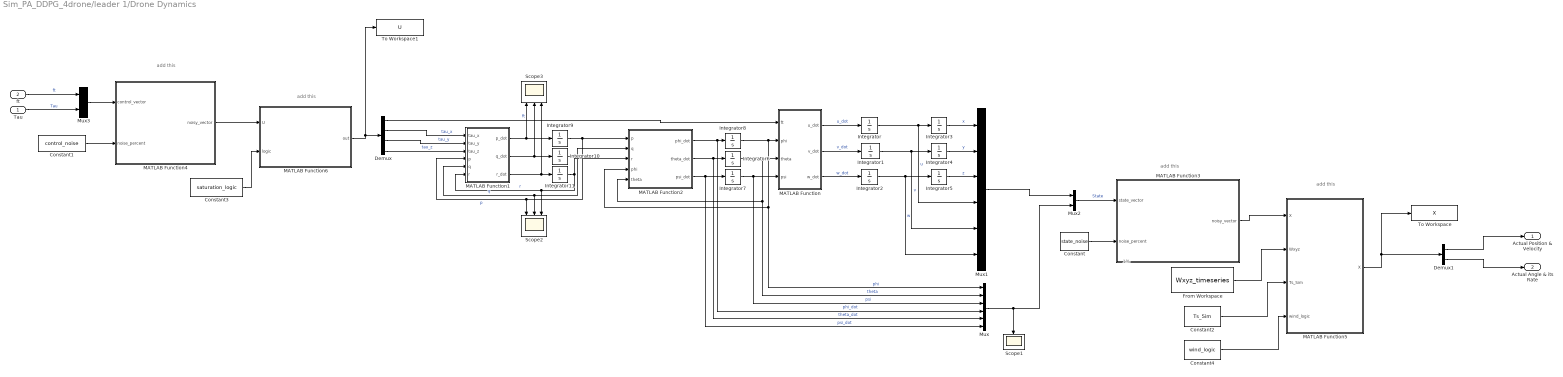
== system Sim_PA_DDPG_4drone/leader 1/Drone Dynamics ==
  note: add this
  note: 1%
  note: add this
  note: add this
  note: add this
  Tau : Inport
  ft : Inport  Port=2
  Constant : Constant  Value=state_noise  SampleTime=Ts_Sim
  Constant1 : Constant  Value=control_noise
  Constant2 : Constant  Value=Ts_Sim
  Constant3 : Constant  Value=saturation_logic  SampleTime=Ts_Sim
  Constant4 : Constant  Value=wind_logic
  Demux : Demux
  Demux1 : Demux  Outputs=2
  From Workspace : FromWorkspace  VariableName=Wxyz_timeseries  SampleTime=Ts_Sim
  Integrator : Integrator  InitialCondition=u_IC  UpperSaturationLimit=uvw_Limit  LowerSaturationLimit=-uvw_Limit
  Integrator1 : Integrator  InitialCondition=v_IC  UpperSaturationLimit=uvw_Limit  LowerSaturationLimit=-uvw_Limit
  Integrator10 : Integrator  InitialCondition=q_IC  UpperSaturationLimit=pqr_Limit  LowerSaturationLimit=-pqr_Limit
  Integrator11 : Integrator  InitialCondition=r_IC  UpperSaturationLimit=pqr_Limit  LowerSaturationLimit=-pqr_Limit
  Integrator2 : Integrator  InitialCondition=w_IC  UpperSaturationLimit=uvw_Limit  LowerSaturationLimit=-uvw_Limit
  Integrator3 : Integrator  InitialCondition=x_IC  UpperSaturationLimit=xy_Limit  LowerSaturationLimit=-xy_Limit
  Integrator4 : Integrator  InitialCondition=y_IC  UpperSaturationLimit=xy_Limit  LowerSaturationLimit=-xy_Limit
  Integrator5 : Integrator  InitialCondition=z_IC  UpperSaturationLimit=z_Limit  LowerSaturationLimit=-z_Limit
  Integrator6 : Integrator  InitialCondition=theta_IC  UpperSaturationLimit=theta_limit  LowerSaturationLimit=-theta_limit  WrappedStateUpperValue=pi/2  WrappedStateLowerValue=-pi/2
  Integrator7 : Integrator  InitialCondition=psi_IC  UpperSaturationLimit=psi_limit  LowerSaturationLimit=-psi_limit
  Integrator8 : Integrator  InitialCondition=phi_IC  UpperSaturationLimit=phi_limit  LowerSaturationLimit=-phi_limit
  Integrator9 : Integrator  InitialCondition=p_IC  UpperSaturationLimit=pqr_Limit  LowerSaturationLimit=-pqr_Limit
  MATLAB Function : MATLAB Function  TreatAsAtomicUnit=on
  MATLAB Function1 : MATLAB Function  TreatAsAtomicUnit=on
  MATLAB Function2 : MATLAB Function  TreatAsAtomicUnit=on
  MATLAB Function3 : MATLAB Function  TreatAsAtomicUnit=on
  MATLAB Function4 : MATLAB Function  TreatAsAtomicUnit=on
  MATLAB Function5 : MATLAB Function  TreatAsAtomicUnit=on
  MATLAB Function6 : MATLAB Function  TreatAsAtomicUnit=on
  Mux : Mux  Inputs=6
  Mux1 : Mux  Inputs=6
  Mux2 : Mux  Inputs=2
  Mux3 : Mux  Inputs=2
  Scope1 : Scope
      settings: ActiveDisplayYMinimum=-0.79782557910284335  ActiveDisplayYMaximum=0.70695961840012789  DataLoggingVariableName=ScopeData2
  Scope2 : Scope  NumInputPorts=3
      settings: ActiveDisplayYMinimum=-0.95183  ActiveDisplayYMaximum=0.89979  DataLoggingVariableName=ScopeData3
  Scope3 : Scope  NumInputPorts=3
      settings: ActiveDisplayYMinimum=-1  ActiveDisplayYMaximum=1  DataLoggingVariableName=ScopeData4
  To Workspace : ToWorkspace  VariableName=X  SampleTime=Ts_Sim
  To Workspace1 : ToWorkspace  VariableName=U  SampleTime=Ts_Sim
  Actual Position & Velocity : Outport
  Actual Angle & its Rate : Outport  Port=2
  wires:
  Integrator4/1 -> Mux1/2  "y"
  MATLAB Function1/3(r_dot) -> Scope3/3, Integrator11/1
  MATLAB Function1/1(p_dot) -> Scope3/1, Integrator9/1
  Integrator3/1 -> Mux1/1  "x"
  Integrator5/1 -> Mux1/3  "z"
  Integrator1/1 -> Mux1/5, Integrator4/1  "v"
  ft/1 -> Mux3/1  "ft"
  Demux/3 -> MATLAB Function1/2(tau_y)  "tau_y"
  Integrator9/1 -> MATLAB Function1/4(p), Scope2/1, MATLAB Function2/1(p)  "p"
  Integrator11/1 -> MATLAB Function1/6(r), Scope2/3, MATLAB Function2/3(r)  "r"
  Integrator2/1 -> Mux1/6, Integrator5/1  "w"
  Integrator/1 -> Mux1/4, Integrator3/1  "u"
  Tau/1 -> Mux3/2  "Tau"
  Integrator7/1 -> Mux/3, MATLAB Function/4(psi)  "psi"
  Integrator8/1 -> Mux/1, MATLAB Function2/4(phi), MATLAB Function/2(phi)  "phi"
  Integrator6/1 -> MATLAB Function/3(theta), Mux/2, MATLAB Function2/5(theta)  "theta"
  Integrator10/1 -> MATLAB Function2/2(q), MATLAB Function1/5(q), Scope2/2  "q"
  Demux/4 -> MATLAB Function1/3(tau_z)  "tau_z"
  Mux/1 -> Scope1/1, Mux2/2
  MATLAB Function/3(w_dot) -> Integrator2/1  "w_dot"
  MATLAB Function/1(u_dot) -> Integrator/1  "u_dot"
  MATLAB Function/2(v_dot) -> Integrator1/1  "v_dot"
  MATLAB Function1/2(q_dot) -> Scope3/2, Integrator10/1
  Demux/2 -> MATLAB Function1/1(tau_x)  "tau_x"
  MATLAB Function2/1(phi_dot) -> Mux/4, Integrator8/1  "phi_dot"
  MATLAB Function2/2(theta_dot) -> Mux/5, Integrator6/1  "theta_dot"
  MATLAB Function2/3(psi_dot) -> Mux/6, Integrator7/1  "psi_dot"
  Mux2/1 -> MATLAB Function3/1(state_vector)  "State"
  MATLAB Function3/1(noisy_vector) -> MATLAB Function5/1("X ")
  Mux1/1 -> Mux2/1
  Constant/1 -> MATLAB Function3/2(noise_percent)
  Mux3/1 -> MATLAB Function4/1(control_vector)
  Constant1/1 -> MATLAB Function4/2(noise_percent)
  MATLAB Function4/1(noisy_vector) -> MATLAB Function6/1(U)
  Demux/1 -> MATLAB Function/1(ft)  "ft"
  From Workspace/1 -> MATLAB Function5/2(Wxyz)
  Demux1/2 -> Actual Angle & its Rate/1
  Demux1/1 -> Actual Position & Velocity/1
  Constant2/1 -> MATLAB Function5/3(Ts_Sim)
  MATLAB Function5/1(X) -> To Workspace/1, Demux1/1
  MATLAB Function6/1(out) -> To Workspace1/1, Demux/1
  Constant3/1 -> MATLAB Function6/2(logic)
  Constant4/1 -> MATLAB Function5/4(wind_logic)

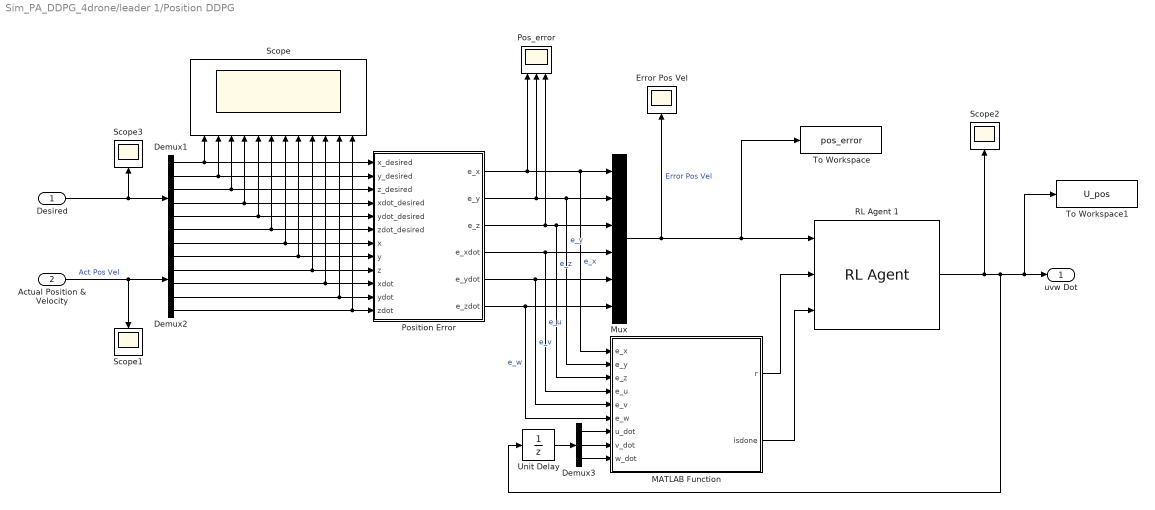
== system Sim_PA_DDPG_4drone/leader 1/Position DDPG ==
  Desired : Inport
  Actual Position & Velocity : Inport  Port=2
  Demux1 : Demux  Outputs=6
  Demux2 : Demux  Outputs=6
  Demux3 : Demux  Outputs=3
  Error Pos Vel : Scope
      settings: ActiveDisplayYMinimum=-20.9607534093343  ActiveDisplayYMaximum=12.051377497018386  DataLoggingVariableName=Error
  MATLAB Function : MATLAB Function  TreatAsAtomicUnit=on
  Mux : Mux  Inputs=6
  Pos_error : Scope  NumInputPorts=3
      settings: ActiveDisplayYMinimum=-21.22024471325139  ActiveDisplayYMaximum=23.007280453639986  DataLoggingVariableName=Error1
  Position Error : MATLAB Function  TreatAsAtomicUnit=on
  RL Agent 1 : rllib/RL Agent  Agent=agent  ExternalActionAsInput=off  ProvideLastAction=off  ProvideCumRwd=off  TreatAsDirectFeedthrough=on  UseStrictObservationDataTypes=off
  Scope : Scope  NumInputPorts=12
      settings: ActiveDisplayYMinimum=-64.8105630976365  ActiveDisplayYMaximum=12.296113517917625  DataLoggingVariableName=Difference
  Scope1 : Scope
      settings: ActiveDisplayYMinimum=-58.848566153955417  ActiveDisplayYMaximum=13.97975040229008  DataLoggingVariableName=Actual
  Scope2 : Scope
      settings: ActiveDisplayYMinimum=-2.3417  ActiveDisplayYMaximum=1.0752  DataLoggingVariableName=ScopeData4
  Scope3 : Scope
      settings: ActiveDisplayYMinimum=-34.036737735877395  ActiveDisplayYMaximum=6.4906396228965306  DataLoggingVariableName=Ref
  To Workspace : ToWorkspace  VariableName=pos_error  SampleTime=Ts_Sim
  To Workspace1 : ToWorkspace  VariableName=U_pos  SampleTime=Ts_Sim
  Unit Delay : UnitDelay  SampleTime=Ts_Sim  HasFrameUpgradeWarning=on
  uvw Dot : Outport
  wires:
  MATLAB Function/1(r) -> RL Agent 1/2
  Mux/1 -> To Workspace/1, RL Agent 1/1, Error Pos Vel/1  "Error Pos Vel"
  RL Agent 1/1 -> To Workspace1/1, uvw Dot/1, Unit Delay/1, Scope2/1
  Position Error/1(e_x) -> MATLAB Function/1(e_x), Mux/1, Pos_error/1  "e_x"
  Position Error/2(e_y) -> MATLAB Function/2(e_y), Mux/2, Pos_error/2  "e_y"
  Position Error/3(e_z) -> Mux/3, MATLAB Function/3(e_z), Pos_error/3  "e_z"
  Position Error/4(e_xdot) -> MATLAB Function/4(e_u), Mux/4  "e_u"
  Position Error/5(e_ydot) -> MATLAB Function/5(e_v), Mux/5  "e_v"
  Position Error/6(e_zdot) -> MATLAB Function/6(e_w), Mux/6  "e_w"
  MATLAB Function/2(isdone) -> RL Agent 1/3
  Demux1/1 -> Position Error/1(x_desired), Scope/1
  Demux1/2 -> Position Error/2(y_desired), Scope/2
  Demux1/3 -> Position Error/3(z_desired), Scope/3
  Demux1/4 -> Position Error/4(xdot_desired), Scope/4
  Demux1/5 -> Position Error/5(ydot_desired), Scope/5
  Demux1/6 -> Position Error/6(zdot_desired), Scope/6
  Desired/1 -> Scope3/1, Demux1/1
  Demux2/1 -> Position Error/7(x), Scope/7
  Demux2/2 -> Position Error/8(y), Scope/8
  Demux2/3 -> Position Error/9(z), Scope/9
  Demux2/4 -> Position Error/10(xdot), Scope/10
  Demux2/5 -> Position Error/11(ydot), Scope/11
  Demux2/6 -> Scope/12, Position Error/12(zdot)
  Actual Position & Velocity/1 -> Demux2/1, Scope1/1  "Act Pos Vel"
  Demux3/1 -> MATLAB Function/7(u_dot)
  Demux3/2 -> MATLAB Function/8(v_dot)
  Demux3/3 -> MATLAB Function/9(w_dot)
  Unit Delay/1 -> Demux3/1

== system Sim_PA_DDPG_4drone/leader 1/System Solver ==
  uvw Dot : Inport
  Clock : Clock
  Constant : Constant  Value=psi_dsr
  Demux : Demux  Outputs=3
  Mux : Mux  Inputs=3
  Scope : Scope
      settings: ActiveDisplayYMinimum=5.5477079741609581  ActiveDisplayYMaximum=13.965080226414941
  System Solver : MATLAB Function  TreatAsAtomicUnit=on
  Ang Ref : Outport
  ft : Outport  Port=2
  wires:
  System Solver/2(pitch) -> Mux/2
  Demux/1 -> System Solver/1(u1)
  System Solver/3(r_yaw) -> Mux/3
  Demux/2 -> System Solver/2(u2)
  System Solver/1(roll) -> Mux/1
  Demux/3 -> System Solver/3(u3)
  System Solver/4(ft) -> ft/1, Scope/1  "ft"
  Clock/1 -> System Solver/4(Ts)
  Mux/1 -> Ang Ref/1  "Ang Ref"
  uvw Dot/1 -> Demux/1
  Constant/1 -> System Solver/5("r_yaw ")

== matlab function Sim_PA_DDPG_4drone/drone 2/Attitude DDPG/Attitude Error ==
  data: phi_dsr input; phi_dot_dsr input; theta_dsr input; theta_dot_dsr input; psi_dsr input; psi_dot_dsr input; phi input; theta input; psi input; e_phi output; e_theta output; e_psi output; phi_dot input; theta_dot input; psi_dot input; e_phi_dot output; e_theta_dot output; e_psi_dot output
function [ e_phi, e_theta, e_psi, e_phi_dot, e_theta_dot, e_psi_dot ] = calculate_errors(phi_dsr, phi_dot_dsr, theta_dsr, theta_dot_dsr, psi_dsr, psi_dot_dsr, phi, theta, psi, phi_dot, theta_dot, psi_dot)
   
    e_phi = phi_dsr - phi;
    e_theta = theta_dsr - theta;
    e_psi = psi_dsr - psi;

    e_phi_dot = phi_dot_dsr - phi_dot;
    e_theta_dot = theta_dot_dsr - theta_dot;
    e_psi_dot = psi_dot_dsr - psi_dot;

end
